simulink model "model_pi"  (R2024b)
settings: Solver=ode113  StartTime=0.0  StopTime=10.0  MaxStep=1e-2  RelTol=1e-3
values from neighbouring files (symbols this model uses):
  A = [A_,zeros(2,1);zeros(1,2),zeros(1,1)]    [run1.m]    (also in run2.m)
  B1 = [B1_;zeros(1,1)]    [run1.m]    (also in run2.m)
  C1 = [C1_,eye(1)]    [run1.m]    (also in run2.m)
  D1 = D1_    [run1.m]    (also in run2.m)
  D2 = D2_    [run1.m]    (also in run2.m)
  L = inv(P)*W    [run1.m]    (also in run2.m)
  x0 = [1;2;3;]    [run1.m]    (also in run2.m)
libraries: simulink x1
settings Model: Creator=mehmetcanevi  LastModifiedBy=mehmetcanevi

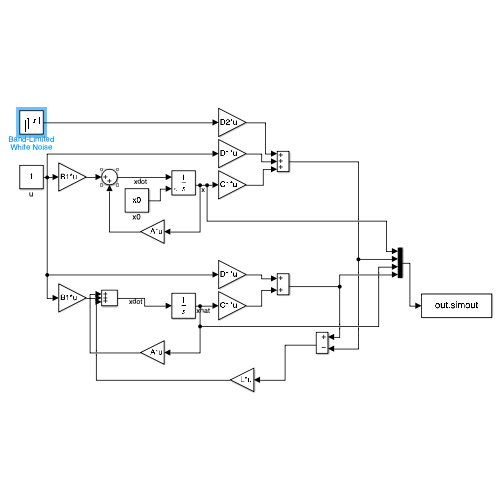
[thumbnail: Simulink's stored preview of the top-level diagram]
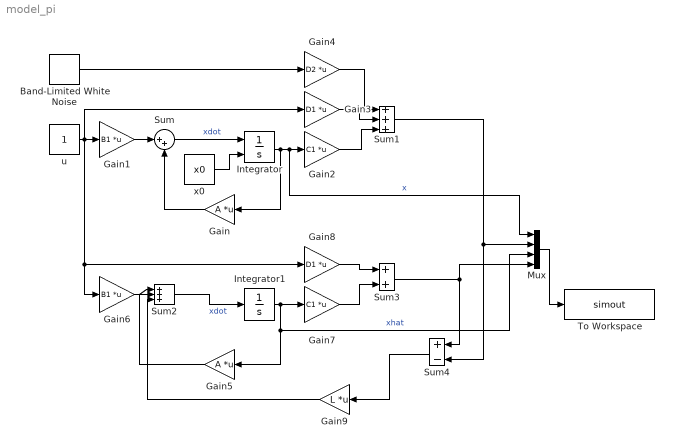
== system model_pi ==
  Band-Limited White Noise : simulink/Sources/Band-Limited White Noise  Cov=[0.001]  Ts=0.1  seed=[23341]
  Gain : Gain  Gain=A  Multiplication=Matrix(K*u)
  Gain1 : Gain  Gain=B1  Multiplication=Matrix(K*u)
  Gain2 : Gain  Gain=C1  Multiplication=Matrix(K*u)
  Gain3 : Gain  Gain=D1  Multiplication=Matrix(K*u)
  Gain4 : Gain  Gain=D2  Multiplication=Matrix(K*u)
  Gain5 : Gain  Gain=A  Multiplication=Matrix(K*u)
  Gain6 : Gain  Gain=B1  Multiplication=Matrix(K*u)
  Gain7 : Gain  Gain=C1  Multiplication=Matrix(K*u)
  Gain8 : Gain  Gain=D1  Multiplication=Matrix(K*u)
  Gain9 : Gain  Gain=L  Multiplication=Matrix(K*u)
  Integrator : Integrator  InitialConditionSource=external
  Integrator1 : Integrator
  Mux : Mux
  Sum : Sum  Inputs=|++
  Sum1 : Sum  Inputs=+++
  Sum2 : Sum  Inputs=+++
  Sum3 : Sum
  Sum4 : Sum  Inputs=+-
  To Workspace : ToWorkspace  VariableName=simout  SampleTime=-1
  u : Constant
  x0 : Constant  Value=x0
  wires:
  Sum/1 -> Integrator/1  "xdot"
  Gain/1 -> Sum/2
  Integrator/1 -> Mux/1, Gain2/1, Gain/1  "x"
  x0/1 -> Integrator/2
  Gain1/1 -> Sum/1
  Gain2/1 -> Sum1/3
  Gain3/1 -> Sum1/2
  Gain4/1 -> Sum1/1
  Band-Limited White Noise/1 -> Gain4/1
  Gain8/1 -> Sum3/1
  Gain7/1 -> Sum3/2
  Gain6/1 -> Sum2/1
  u/1 -> Gain6/1, Gain8/1, Gain3/1, Gain1/1
  Integrator1/1 -> Gain5/1, Mux/3, Gain7/1  "xhat"
  Gain5/1 -> Sum2/2
  Sum2/1 -> Integrator1/1  "xdot"
  Gain9/1 -> Sum2/3
  Sum3/1 -> Sum4/1, Mux/4
  Sum1/1 -> Mux/2, Sum4/2
  Sum4/1 -> Gain9/1
  Mux/1 -> To Workspace/1
